simulink model "nn_plus"  (R2018b)
settings: Solver=VariableStepAuto  StartTime=0.0  StopTime=10.0  RelTol=1e-3
libraries: neural x265
(part 1 of 2)
settings Model: Creator=Mihail  LastModifiedBy=Mihail

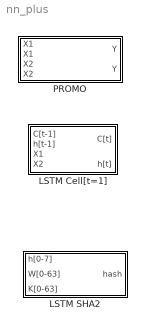
== system nn_plus ==
  LSTM Cell[t=1] : Subsystem
  LSTM SHA2 : Subsystem
  PROMO : Subsystem

== system nn_plus/LSTM Cell[t=1] ==
  note: LSTM Cell L1 (Block-Scheme)
  C[t-1] : Inport
  h[t-1] : Inport  Port=2
  X1 : Inport  Port=3
  X2 : Inport  Port=4
  Product : Product
  Product1 : Product
  Sum : Sum  Inputs=|++
  Sum1 : Sum  Inputs=|++
  Vector Concatenate : Concatenate  NumInputs=3
  logsig : neural/Transfer Functions/logsig
  logsig1 : neural/Transfer Functions/logsig
  logsig2 : neural/Transfer Functions/logsig
  tansig3 : neural/Transfer Functions/tansig
  tansig4 : neural/Transfer Functions/tansig
  C[t] : Outport
  h[t] : Outport  Port=2
  wires:
  h[t-1]/1 -> Vector Concatenate/1
  X1/1 -> Vector Concatenate/2
  X2/1 -> Vector Concatenate/3
  Vector Concatenate/1 -> logsig/1, logsig2/1, tansig3/1, logsig1/1
  C[t-1]/1 -> Sum/1
  logsig/1 -> Sum/2
  Sum/1 -> Sum1/1
  tansig3/1 -> Product/2
  logsig1/1 -> Product/1
  Product/1 -> Sum1/2
  logsig2/1 -> Product1/2
  Sum1/1 -> C[t]/1, tansig4/1
  tansig4/1 -> Product1/1
  Product1/1 -> h[t]/1

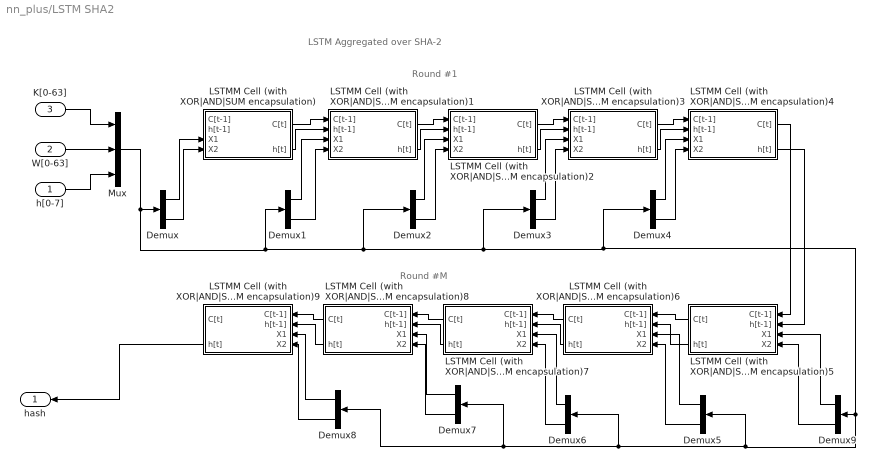
== system nn_plus/LSTM SHA2 ==
  note: Round #M
  note: Round #1
  note: LSTM Aggregated over SHA-2
  h[0-7] : Inport
  W[0-63] : Inport  Port=2
  K[0-63] : Inport  Port=3
  Demux{,1..9} (10 alike) : Demux  Outputs=2
  LSTMM Cell (with XOR|AND|SUM encapsulation) : Subsystem
  LSTMM Cell (with XOR|AND|SUM encapsulation)1 : Subsystem
  LSTMM Cell (with XOR|AND|SUM encapsulation)2 : Subsystem
  LSTMM Cell (with XOR|AND|SUM encapsulation)3 : Subsystem
  LSTMM Cell (with XOR|AND|SUM encapsulation)4 : Subsystem
  LSTMM Cell (with XOR|AND|SUM encapsulation)5 : Subsystem
  LSTMM Cell (with XOR|AND|SUM encapsulation)6 : Subsystem
  LSTMM Cell (with XOR|AND|SUM encapsulation)7 : Subsystem
  LSTMM Cell (with XOR|AND|SUM encapsulation)8 : Subsystem
  LSTMM Cell (with XOR|AND|SUM encapsulation)9 : Subsystem
  Mux : Mux  Inputs=3
  hash : Outport
  wires:
  Mux/1 -> Demux8/1, Demux7/1, Demux6/1, Demux5/1, Demux9/1, Demux4/1, Demux3/1, Demux2/1, Demux1/1, Demux/1
  Demux9/2 -> LSTMM Cell (with XOR|AND|SUM encapsulation)5/4(X2)
  LSTMM Cell (with XOR|AND|SUM encapsulation)7/2(h[t]) -> LSTMM Cell (with XOR|AND|SUM encapsulation)8/2(h[t-1])
  LSTMM Cell (with XOR|AND|SUM encapsulation)8/1(C[t]) -> LSTMM Cell (with XOR|AND|SUM encapsulation)9/1(C[t-1])
  LSTMM Cell (with XOR|AND|SUM encapsulation)5/2(h[t]) -> LSTMM Cell (with XOR|AND|SUM encapsulation)6/2(h[t-1])
  Demux5/1 -> LSTMM Cell (with XOR|AND|SUM encapsulation)6/3(X1)
  LSTMM Cell (with XOR|AND|SUM encapsulation)7/1(C[t]) -> LSTMM Cell (with XOR|AND|SUM encapsulation)8/1(C[t-1])
  Demux2/2 -> LSTMM Cell (with XOR|AND|SUM encapsulation)2/4(X2)
  Demux1/2 -> LSTMM Cell (with XOR|AND|SUM encapsulation)1/4(X2)
  Demux2/1 -> LSTMM Cell (with XOR|AND|SUM encapsulation)2/3(X1)
  Demux4/2 -> LSTMM Cell (with XOR|AND|SUM encapsulation)4/4(X2)
  Demux4/1 -> LSTMM Cell (with XOR|AND|SUM encapsulation)4/3(X1)
  Demux3/2 -> LSTMM Cell (with XOR|AND|SUM encapsulation)3/4(X2)
  Demux3/1 -> LSTMM Cell (with XOR|AND|SUM encapsulation)3/3(X1)
  Demux1/1 -> LSTMM Cell (with XOR|AND|SUM encapsulation)1/3(X1)
  LSTMM Cell (with XOR|AND|SUM encapsulation)2/2(h[t]) -> LSTMM Cell (with XOR|AND|SUM encapsulation)3/2(h[t-1])
  Demux7/1 -> LSTMM Cell (with XOR|AND|SUM encapsulation)8/3(X1)
  Demux/1 -> LSTMM Cell (with XOR|AND|SUM encapsulation)/3(X1)
  LSTMM Cell (with XOR|AND|SUM encapsulation)2/1(C[t]) -> LSTMM Cell (with XOR|AND|SUM encapsulation)3/1(C[t-1])
  Demux9/1 -> LSTMM Cell (with XOR|AND|SUM encapsulation)5/3(X1)
  Demux6/1 -> LSTMM Cell (with XOR|AND|SUM encapsulation)7/3(X1)
  Demux8/1 -> LSTMM Cell (with XOR|AND|SUM encapsulation)9/3(X1)
  Demux5/2 -> LSTMM Cell (with XOR|AND|SUM encapsulation)6/4(X2)
  Demux8/2 -> LSTMM Cell (with XOR|AND|SUM encapsulation)9/4(X2)
  LSTMM Cell (with XOR|AND|SUM encapsulation)8/2(h[t]) -> LSTMM Cell (with XOR|AND|SUM encapsulation)9/2(h[t-1])
  Demux7/2 -> LSTMM Cell (with XOR|AND|SUM encapsulation)8/4(X2)
  LSTMM Cell (with XOR|AND|SUM encapsulation)6/2(h[t]) -> LSTMM Cell (with XOR|AND|SUM encapsulation)7/2(h[t-1])
  Demux/2 -> LSTMM Cell (with XOR|AND|SUM encapsulation)/4(X2)
  K[0-63]/1 -> Mux/1
  LSTMM Cell (with XOR|AND|SUM encapsulation)/2(h[t]) -> LSTMM Cell (with XOR|AND|SUM encapsulation)1/2(h[t-1])
  LSTMM Cell (with XOR|AND|SUM encapsulation)1/2(h[t]) -> LSTMM Cell (with XOR|AND|SUM encapsulation)2/2(h[t-1])
  LSTMM Cell (with XOR|AND|SUM encapsulation)1/1(C[t]) -> LSTMM Cell (with XOR|AND|SUM encapsulation)2/1(C[t-1])
  LSTMM Cell (with XOR|AND|SUM encapsulation)9/2(h[t]) -> hash/1
  LSTMM Cell (with XOR|AND|SUM encapsulation)/1(C[t]) -> LSTMM Cell (with XOR|AND|SUM encapsulation)1/1(C[t-1])
  LSTMM Cell (with XOR|AND|SUM encapsulation)6/1(C[t]) -> LSTMM Cell (with XOR|AND|SUM encapsulation)7/1(C[t-1])
  LSTMM Cell (with XOR|AND|SUM encapsulation)3/1(C[t]) -> LSTMM Cell (with XOR|AND|SUM encapsulation)4/1(C[t-1])
  LSTMM Cell (with XOR|AND|SUM encapsulation)4/1(C[t]) -> LSTMM Cell (with XOR|AND|SUM encapsulation)5/1(C[t-1])
  W[0-63]/1 -> Mux/2
  Demux6/2 -> LSTMM Cell (with XOR|AND|SUM encapsulation)7/4(X2)
  LSTMM Cell (with XOR|AND|SUM encapsulation)4/2(h[t]) -> LSTMM Cell (with XOR|AND|SUM encapsulation)5/2(h[t-1])
  LSTMM Cell (with XOR|AND|SUM encapsulation)3/2(h[t]) -> LSTMM Cell (with XOR|AND|SUM encapsulation)4/2(h[t-1])
  h[0-7]/1 -> Mux/3
  LSTMM Cell (with XOR|AND|SUM encapsulation)5/1(C[t]) -> LSTMM Cell (with XOR|AND|SUM encapsulation)6/1(C[t-1])

== system nn_plus/PROMO ==
  note: SUM Overloaded
      | (Block-Scheme)
  note: SUM (As displayed)
  "X1 " : Inport
  X1 : Inport  Port=2
  X2 : Inport  Port=3
  "X2 " : Inport  Port=4
  Demux : Demux  Outputs=32
  Demux1 : Demux  Outputs=32
  Mux : Mux  Inputs=32
  SUM NN : Subsystem
  Sum : Sum  Inputs=|++
  Y : Outport
  "Y " : Outport  Port=2
  wires:
  Demux1/3 -> SUM NN/4(X2[t=1])
  Demux/32 -> SUM NN/7(X1[t=31])
  SUM NN/2(Y[t=1]) -> Mux/2
  SUM NN/1(Y[t=0]) -> Mux/1
  Demux/3 -> SUM NN/3(X1[t=1])
  Demux1/2 -> SUM NN/2(X2[t=0])
  SUM NN/4(Y[t=31]) -> Mux/32
  Demux1/32 -> SUM NN/8(X2[t=31])
  X1/1 -> Demux/1
  X2/1 -> Demux1/1
  "X2 "/1 -> Sum/2
  Sum/1 -> "Y "/1
  Mux/1 -> Y/1
  Demux/2 -> SUM NN/1(X1[t=0])
  "X1 "/1 -> Sum/1
  SUM NN/3(Y[t]) -> Mux/19

== system nn_plus/LSTM SHA2/LSTMM Cell (with XOR|AND|SUM encapsulation) ==
  note: LSTM Cell with LSTMM | XOR | AND NN (Used As Activation)
  C[t-1] : Inport
  h[t-1] : Inport  Port=2
  X1 : Inport  Port=3
  X2 : Inport  Port=4
  Demux : Demux  Outputs=2
  LSTM | XOR |AND (NN) : Subsystem
  Product : Product
  Product1 : Product
  Sum : Sum  Inputs=|++
  Sum1 : Sum  Inputs=|++
  Vector Concatenate : Concatenate  NumInputs=3
  logsig : neural/Transfer Functions/logsig
  logsig1 : neural/Transfer Functions/logsig
  tansig3 : neural/Transfer Functions/tansig
  tansig4 : neural/Transfer Functions/tansig
  C[t] : Outport
  h[t] : Outport  Port=2
  wires:
  h[t-1]/1 -> Vector Concatenate/1
  X1/1 -> Vector Concatenate/2
  X2/1 -> Vector Concatenate/3
  Vector Concatenate/1 -> logsig/1, Demux/1, tansig3/1, logsig1/1
  C[t-1]/1 -> Sum/1
  logsig/1 -> Sum/2
  Sum/1 -> Sum1/1
  tansig3/1 -> Product/2
  logsig1/1 -> Product/1
  Product/1 -> Sum1/2
  Sum1/1 -> C[t]/1, tansig4/1
  tansig4/1 -> Product1/1
  Product1/1 -> h[t]/1
  Demux/1 -> LSTM | XOR |AND (NN)/1(X1)
  Demux/2 -> LSTM | XOR |AND (NN)/2(X2)
  LSTM | XOR |AND (NN)/1(Y) -> Product1/2

== system nn_plus/LSTM SHA2/LSTMM Cell (with XOR|AND|SUM encapsulation)1 ==
  note: LSTM Cell with LSTMM | XOR | AND NN (Used As Activation)
  C[t-1] : Inport
  h[t-1] : Inport  Port=2
  X1 : Inport  Port=3
  X2 : Inport  Port=4
  Demux : Demux  Outputs=2
  LSTM | XOR |AND (NN) : Subsystem
  Product : Product
  Product1 : Product
  Sum : Sum  Inputs=|++
  Sum1 : Sum  Inputs=|++
  Vector Concatenate : Concatenate  NumInputs=3
  logsig : neural/Transfer Functions/logsig
  logsig1 : neural/Transfer Functions/logsig
  tansig3 : neural/Transfer Functions/tansig
  tansig4 : neural/Transfer Functions/tansig
  C[t] : Outport
  h[t] : Outport  Port=2
  wires:
  h[t-1]/1 -> Vector Concatenate/1
  X1/1 -> Vector Concatenate/2
  X2/1 -> Vector Concatenate/3
  Vector Concatenate/1 -> logsig/1, Demux/1, tansig3/1, logsig1/1
  C[t-1]/1 -> Sum/1
  logsig/1 -> Sum/2
  Sum/1 -> Sum1/1
  tansig3/1 -> Product/2
  logsig1/1 -> Product/1
  Product/1 -> Sum1/2
  Sum1/1 -> C[t]/1, tansig4/1
  tansig4/1 -> Product1/1
  Product1/1 -> h[t]/1
  Demux/1 -> LSTM | XOR |AND (NN)/1(X1)
  Demux/2 -> LSTM | XOR |AND (NN)/2(X2)
  LSTM | XOR |AND (NN)/1(Y) -> Product1/2

== system nn_plus/LSTM SHA2/LSTMM Cell (with XOR|AND|SUM encapsulation)2 ==
  note: LSTM Cell with LSTMM | XOR | AND NN (Used As Activation)
  C[t-1] : Inport
  h[t-1] : Inport  Port=2
  X1 : Inport  Port=3
  X2 : Inport  Port=4
  Demux : Demux  Outputs=2
  LSTM | XOR |AND (NN) : Subsystem
  Product : Product
  Product1 : Product
  Sum : Sum  Inputs=|++
  Sum1 : Sum  Inputs=|++
  Vector Concatenate : Concatenate  NumInputs=3
  logsig : neural/Transfer Functions/logsig
  logsig1 : neural/Transfer Functions/logsig
  tansig3 : neural/Transfer Functions/tansig
  tansig4 : neural/Transfer Functions/tansig
  C[t] : Outport
  h[t] : Outport  Port=2
  wires:
  h[t-1]/1 -> Vector Concatenate/1
  X1/1 -> Vector Concatenate/2
  X2/1 -> Vector Concatenate/3
  Vector Concatenate/1 -> logsig/1, Demux/1, tansig3/1, logsig1/1
  C[t-1]/1 -> Sum/1
  logsig/1 -> Sum/2
  Sum/1 -> Sum1/1
  tansig3/1 -> Product/2
  logsig1/1 -> Product/1
  Product/1 -> Sum1/2
  Sum1/1 -> C[t]/1, tansig4/1
  tansig4/1 -> Product1/1
  Product1/1 -> h[t]/1
  Demux/1 -> LSTM | XOR |AND (NN)/1(X1)
  Demux/2 -> LSTM | XOR |AND (NN)/2(X2)
  LSTM | XOR |AND (NN)/1(Y) -> Product1/2

== system nn_plus/LSTM SHA2/LSTMM Cell (with XOR|AND|SUM encapsulation)3 ==
  note: LSTM Cell with LSTMM | XOR | AND NN (Used As Activation)
  C[t-1] : Inport
  h[t-1] : Inport  Port=2
  X1 : Inport  Port=3
  X2 : Inport  Port=4
  Demux : Demux  Outputs=2
  LSTM | XOR |AND (NN) : Subsystem
  Product : Product
  Product1 : Product
  Sum : Sum  Inputs=|++
  Sum1 : Sum  Inputs=|++
  Vector Concatenate : Concatenate  NumInputs=3
  logsig : neural/Transfer Functions/logsig
  logsig1 : neural/Transfer Functions/logsig
  tansig3 : neural/Transfer Functions/tansig
  tansig4 : neural/Transfer Functions/tansig
  C[t] : Outport
  h[t] : Outport  Port=2
  wires:
  h[t-1]/1 -> Vector Concatenate/1
  X1/1 -> Vector Concatenate/2
  X2/1 -> Vector Concatenate/3
  Vector Concatenate/1 -> logsig/1, Demux/1, tansig3/1, logsig1/1
  C[t-1]/1 -> Sum/1
  logsig/1 -> Sum/2
  Sum/1 -> Sum1/1
  tansig3/1 -> Product/2
  logsig1/1 -> Product/1
  Product/1 -> Sum1/2
  Sum1/1 -> C[t]/1, tansig4/1
  tansig4/1 -> Product1/1
  Product1/1 -> h[t]/1
  Demux/1 -> LSTM | XOR |AND (NN)/1(X1)
  Demux/2 -> LSTM | XOR |AND (NN)/2(X2)
  LSTM | XOR |AND (NN)/1(Y) -> Product1/2

== system nn_plus/LSTM SHA2/LSTMM Cell (with XOR|AND|SUM encapsulation)4 ==
  note: LSTM Cell with LSTMM | XOR | AND NN (Used As Activation)
  C[t-1] : Inport
  h[t-1] : Inport  Port=2
  X1 : Inport  Port=3
  X2 : Inport  Port=4
  Demux : Demux  Outputs=2
  LSTM | XOR |AND (NN) : Subsystem
  Product : Product
  Product1 : Product
  Sum : Sum  Inputs=|++
  Sum1 : Sum  Inputs=|++
  Vector Concatenate : Concatenate  NumInputs=3
  logsig : neural/Transfer Functions/logsig
  logsig1 : neural/Transfer Functions/logsig
  tansig3 : neural/Transfer Functions/tansig
  tansig4 : neural/Transfer Functions/tansig
  C[t] : Outport
  h[t] : Outport  Port=2
  wires:
  h[t-1]/1 -> Vector Concatenate/1
  X1/1 -> Vector Concatenate/2
  X2/1 -> Vector Concatenate/3
  Vector Concatenate/1 -> logsig/1, Demux/1, tansig3/1, logsig1/1
  C[t-1]/1 -> Sum/1
  logsig/1 -> Sum/2
  Sum/1 -> Sum1/1
  tansig3/1 -> Product/2
  logsig1/1 -> Product/1
  Product/1 -> Sum1/2
  Sum1/1 -> C[t]/1, tansig4/1
  tansig4/1 -> Product1/1
  Product1/1 -> h[t]/1
  Demux/1 -> LSTM | XOR |AND (NN)/1(X1)
  Demux/2 -> LSTM | XOR |AND (NN)/2(X2)
  LSTM | XOR |AND (NN)/1(Y) -> Product1/2

== system nn_plus/LSTM SHA2/LSTMM Cell (with XOR|AND|SUM encapsulation)5 ==
  note: LSTM Cell with LSTMM | XOR | AND NN (Used As Activation)
  C[t-1] : Inport
  h[t-1] : Inport  Port=2
  X1 : Inport  Port=3
  X2 : Inport  Port=4
  Demux : Demux  Outputs=2
  LSTM | XOR |AND (NN) : Subsystem
  Product : Product
  Product1 : Product
  Sum : Sum  Inputs=|++
  Sum1 : Sum  Inputs=|++
  Vector Concatenate : Concatenate  NumInputs=3
  logsig : neural/Transfer Functions/logsig
  logsig1 : neural/Transfer Functions/logsig
  tansig3 : neural/Transfer Functions/tansig
  tansig4 : neural/Transfer Functions/tansig
  C[t] : Outport
  h[t] : Outport  Port=2
  wires:
  h[t-1]/1 -> Vector Concatenate/1
  X1/1 -> Vector Concatenate/2
  X2/1 -> Vector Concatenate/3
  Vector Concatenate/1 -> logsig/1, Demux/1, tansig3/1, logsig1/1
  C[t-1]/1 -> Sum/1
  logsig/1 -> Sum/2
  Sum/1 -> Sum1/1
  tansig3/1 -> Product/2
  logsig1/1 -> Product/1
  Product/1 -> Sum1/2
  Sum1/1 -> C[t]/1, tansig4/1
  tansig4/1 -> Product1/1
  Product1/1 -> h[t]/1
  Demux/1 -> LSTM | XOR |AND (NN)/1(X1)
  Demux/2 -> LSTM | XOR |AND (NN)/2(X2)
  LSTM | XOR |AND (NN)/1(Y) -> Product1/2

== system nn_plus/LSTM SHA2/LSTMM Cell (with XOR|AND|SUM encapsulation)6 ==
  note: LSTM Cell with LSTMM | XOR | AND NN (Used As Activation)
  C[t-1] : Inport
  h[t-1] : Inport  Port=2
  X1 : Inport  Port=3
  X2 : Inport  Port=4
  Demux : Demux  Outputs=2
  LSTM | XOR |AND (NN) : Subsystem
  Product : Product
  Product1 : Product
  Sum : Sum  Inputs=|++
  Sum1 : Sum  Inputs=|++
  Vector Concatenate : Concatenate  NumInputs=3
  logsig : neural/Transfer Functions/logsig
  logsig1 : neural/Transfer Functions/logsig
  tansig3 : neural/Transfer Functions/tansig
  tansig4 : neural/Transfer Functions/tansig
  C[t] : Outport
  h[t] : Outport  Port=2
  wires:
  h[t-1]/1 -> Vector Concatenate/1
  X1/1 -> Vector Concatenate/2
  X2/1 -> Vector Concatenate/3
  Vector Concatenate/1 -> logsig/1, Demux/1, tansig3/1, logsig1/1
  C[t-1]/1 -> Sum/1
  logsig/1 -> Sum/2
  Sum/1 -> Sum1/1
  tansig3/1 -> Product/2
  logsig1/1 -> Product/1
  Product/1 -> Sum1/2
  Sum1/1 -> C[t]/1, tansig4/1
  tansig4/1 -> Product1/1
  Product1/1 -> h[t]/1
  Demux/1 -> LSTM | XOR |AND (NN)/1(X1)
  Demux/2 -> LSTM | XOR |AND (NN)/2(X2)
  LSTM | XOR |AND (NN)/1(Y) -> Product1/2

== system nn_plus/LSTM SHA2/LSTMM Cell (with XOR|AND|SUM encapsulation)7 ==
  note: LSTM Cell with LSTMM | XOR | AND NN (Used As Activation)
  C[t-1] : Inport
  h[t-1] : Inport  Port=2
  X1 : Inport  Port=3
  X2 : Inport  Port=4
  Demux : Demux  Outputs=2
  LSTM | XOR |AND (NN) : Subsystem
  Product : Product
  Product1 : Product
  Sum : Sum  Inputs=|++
  Sum1 : Sum  Inputs=|++
  Vector Concatenate : Concatenate  NumInputs=3
  logsig : neural/Transfer Functions/logsig
  logsig1 : neural/Transfer Functions/logsig
  tansig3 : neural/Transfer Functions/tansig
  tansig4 : neural/Transfer Functions/tansig
  C[t] : Outport
  h[t] : Outport  Port=2
  wires:
  h[t-1]/1 -> Vector Concatenate/1
  X1/1 -> Vector Concatenate/2
  X2/1 -> Vector Concatenate/3
  Vector Concatenate/1 -> logsig/1, Demux/1, tansig3/1, logsig1/1
  C[t-1]/1 -> Sum/1
  logsig/1 -> Sum/2
  Sum/1 -> Sum1/1
  tansig3/1 -> Product/2
  logsig1/1 -> Product/1
  Product/1 -> Sum1/2
  Sum1/1 -> C[t]/1, tansig4/1
  tansig4/1 -> Product1/1
  Product1/1 -> h[t]/1
  Demux/1 -> LSTM | XOR |AND (NN)/1(X1)
  Demux/2 -> LSTM | XOR |AND (NN)/2(X2)
  LSTM | XOR |AND (NN)/1(Y) -> Product1/2

== system nn_plus/LSTM SHA2/LSTMM Cell (with XOR|AND|SUM encapsulation)8 ==
  note: LSTM Cell with LSTMM | XOR | AND NN (Used As Activation)
  C[t-1] : Inport
  h[t-1] : Inport  Port=2
  X1 : Inport  Port=3
  X2 : Inport  Port=4
  Demux : Demux  Outputs=2
  LSTM | XOR |AND (NN) : Subsystem
  Product : Product
  Product1 : Product
  Sum : Sum  Inputs=|++
  Sum1 : Sum  Inputs=|++
  Vector Concatenate : Concatenate  NumInputs=3
  logsig : neural/Transfer Functions/logsig
  logsig1 : neural/Transfer Functions/logsig
  tansig3 : neural/Transfer Functions/tansig
  tansig4 : neural/Transfer Functions/tansig
  C[t] : Outport
  h[t] : Outport  Port=2
  wires:
  h[t-1]/1 -> Vector Concatenate/1
  X1/1 -> Vector Concatenate/2
  X2/1 -> Vector Concatenate/3
  Vector Concatenate/1 -> logsig/1, Demux/1, tansig3/1, logsig1/1
  C[t-1]/1 -> Sum/1
  logsig/1 -> Sum/2
  Sum/1 -> Sum1/1
  tansig3/1 -> Product/2
  logsig1/1 -> Product/1
  Product/1 -> Sum1/2
  Sum1/1 -> C[t]/1, tansig4/1
  tansig4/1 -> Product1/1
  Product1/1 -> h[t]/1
  Demux/1 -> LSTM | XOR |AND (NN)/1(X1)
  Demux/2 -> LSTM | XOR |AND (NN)/2(X2)
  LSTM | XOR |AND (NN)/1(Y) -> Product1/2

== system nn_plus/LSTM SHA2/LSTMM Cell (with XOR|AND|SUM encapsulation)9 ==
  note: LSTM Cell with LSTMM | XOR | AND NN (Used As Activation)
  C[t-1] : Inport
  h[t-1] : Inport  Port=2
  X1 : Inport  Port=3
  X2 : Inport  Port=4
  Demux : Demux  Outputs=2
  LSTM | XOR |AND (NN) : Subsystem
  Product : Product
  Product1 : Product
  Sum : Sum  Inputs=|++
  Sum1 : Sum  Inputs=|++
  Vector Concatenate : Concatenate  NumInputs=3
  logsig : neural/Transfer Functions/logsig
  logsig1 : neural/Transfer Functions/logsig
  tansig3 : neural/Transfer Functions/tansig
  tansig4 : neural/Transfer Functions/tansig
  C[t] : Outport
  h[t] : Outport  Port=2
  wires:
  h[t-1]/1 -> Vector Concatenate/1
  X1/1 -> Vector Concatenate/2
  X2/1 -> Vector Concatenate/3
  Vector Concatenate/1 -> logsig/1, Demux/1, tansig3/1, logsig1/1
  C[t-1]/1 -> Sum/1
  logsig/1 -> Sum/2
  Sum/1 -> Sum1/1
  tansig3/1 -> Product/2
  logsig1/1 -> Product/1
  Product/1 -> Sum1/2
  Sum1/1 -> C[t]/1, tansig4/1
  tansig4/1 -> Product1/1
  Product1/1 -> h[t]/1
  Demux/1 -> LSTM | XOR |AND (NN)/1(X1)
  Demux/2 -> LSTM | XOR |AND (NN)/2(X2)
  LSTM | XOR |AND (NN)/1(Y) -> Product1/2

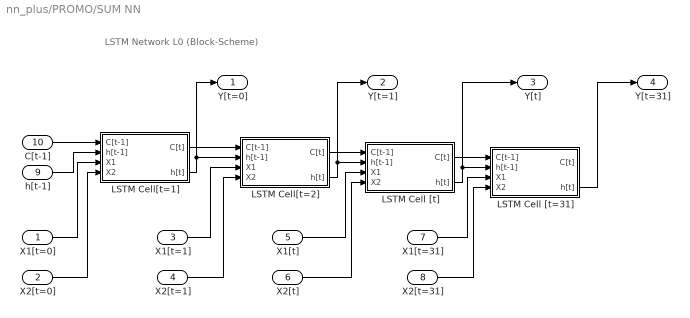
== system nn_plus/PROMO/SUM NN ==
  note: LSTM Network L0 (Block-Scheme)
  X1[t=0] : Inport
  X2[t=0] : Inport  Port=2
  X1[t=1] : Inport  Port=3
  X2[t=1] : Inport  Port=4
  X1[t] : Inport  Port=5
  X2[t] : Inport  Port=6
  X1[t=31] : Inport  Port=7
  X2[t=31] : Inport  Port=8
  h[t-1] : Inport  Port=9
  C[t-1] : Inport  Port=10
  LSTM Cell [t=31] : Subsystem
  LSTM Cell [t] : Subsystem
  LSTM Cell[t=1] : Subsystem
  LSTM Cell[t=2] : Subsystem
  Y[t=0] : Outport
  Y[t=1] : Outport  Port=2
  Y[t] : Outport  Port=3
  Y[t=31] : Outport  Port=4
  wires:
  C[t-1]/1 -> LSTM Cell[t=1]/1(C[t-1])
  h[t-1]/1 -> LSTM Cell[t=1]/2(h[t-1])
  LSTM Cell[t=1]/1(C[t]) -> LSTM Cell[t=2]/1(C[t-1])
  LSTM Cell[t=1]/2(h[t]) -> Y[t=0]/1, LSTM Cell[t=2]/2(h[t-1])
  X1[t=0]/1 -> LSTM Cell[t=1]/3(X1)
  X2[t=0]/1 -> LSTM Cell[t=1]/4(X2)
  X1[t=1]/1 -> LSTM Cell[t=2]/3(X1)
  X2[t=1]/1 -> LSTM Cell[t=2]/4(X2)
  LSTM Cell[t=2]/1(C[t]) -> LSTM Cell [t]/1(C[t-1])
  LSTM Cell[t=2]/2(h[t]) -> Y[t=1]/1, LSTM Cell [t]/2(h[t-1])
  LSTM Cell [t]/1(C[t]) -> LSTM Cell [t=31]/1(C[t-1])
  X2[t]/1 -> LSTM Cell [t]/4(X2)
  X1[t]/1 -> LSTM Cell [t]/3(X1)
  X1[t=31]/1 -> LSTM Cell [t=31]/3(X1)
  X2[t=31]/1 -> LSTM Cell [t=31]/4(X2)
  LSTM Cell [t=31]/2(h[t]) -> Y[t=31]/1
  LSTM Cell [t]/2(h[t]) -> Y[t]/1, LSTM Cell [t=31]/2(h[t-1])

== system nn_plus/LSTM SHA2/LSTMM Cell (with XOR|AND|SUM encapsulation)/LSTM | XOR |AND (NN) ==
  note: SUM Overloaded
      | (Block-Scheme)
  X1 : Inport
  X2 : Inport  Port=2
  Demux : Demux  Outputs=32
  Demux1 : Demux  Outputs=32
  Mux : Mux  Inputs=32
  SUM NN : Subsystem
  Y : Outport
  wires:
  Demux1/3 -> SUM NN/4(X2[t=1])
  Demux/32 -> SUM NN/7(X1[t=31])
  SUM NN/2(Y[t=1]) -> Mux/2
  SUM NN/1(Y[t=0]) -> Mux/1
  Demux/3 -> SUM NN/3(X1[t=1])
  Demux1/2 -> SUM NN/2(X2[t=0])
  SUM NN/4(Y[t=31]) -> Mux/32
  Demux1/32 -> SUM NN/8(X2[t=31])
  X1/1 -> Demux/1
  X2/1 -> Demux1/1
  Mux/1 -> Y/1
  Demux/2 -> SUM NN/1(X1[t=0])
  SUM NN/3(Y[t]) -> Mux/19

== system nn_plus/LSTM SHA2/LSTMM Cell (with XOR|AND|SUM encapsulation)1/LSTM | XOR |AND (NN) ==
  note: SUM Overloaded
      | (Block-Scheme)
  X1 : Inport
  X2 : Inport  Port=2
  Demux : Demux  Outputs=32
  Demux1 : Demux  Outputs=32
  Mux : Mux  Inputs=32
  SUM NN : Subsystem
  Y : Outport
  wires:
  Demux1/3 -> SUM NN/4(X2[t=1])
  Demux/32 -> SUM NN/7(X1[t=31])
  SUM NN/2(Y[t=1]) -> Mux/2
  SUM NN/1(Y[t=0]) -> Mux/1
  Demux/3 -> SUM NN/3(X1[t=1])
  Demux1/2 -> SUM NN/2(X2[t=0])
  SUM NN/4(Y[t=31]) -> Mux/32
  Demux1/32 -> SUM NN/8(X2[t=31])
  X1/1 -> Demux/1
  X2/1 -> Demux1/1
  Mux/1 -> Y/1
  Demux/2 -> SUM NN/1(X1[t=0])
  SUM NN/3(Y[t]) -> Mux/19

== system nn_plus/LSTM SHA2/LSTMM Cell (with XOR|AND|SUM encapsulation)2/LSTM | XOR |AND (NN) ==
  note: SUM Overloaded
      | (Block-Scheme)
  X1 : Inport
  X2 : Inport  Port=2
  Demux : Demux  Outputs=32
  Demux1 : Demux  Outputs=32
  Mux : Mux  Inputs=32
  SUM NN : Subsystem
  Y : Outport
  wires:
  Demux1/3 -> SUM NN/4(X2[t=1])
  Demux/32 -> SUM NN/7(X1[t=31])
  SUM NN/2(Y[t=1]) -> Mux/2
  SUM NN/1(Y[t=0]) -> Mux/1
  Demux/3 -> SUM NN/3(X1[t=1])
  Demux1/2 -> SUM NN/2(X2[t=0])
  SUM NN/4(Y[t=31]) -> Mux/32
  Demux1/32 -> SUM NN/8(X2[t=31])
  X1/1 -> Demux/1
  X2/1 -> Demux1/1
  Mux/1 -> Y/1
  Demux/2 -> SUM NN/1(X1[t=0])
  SUM NN/3(Y[t]) -> Mux/19

== system nn_plus/LSTM SHA2/LSTMM Cell (with XOR|AND|SUM encapsulation)3/LSTM | XOR |AND (NN) ==
  note: SUM Overloaded
      | (Block-Scheme)
  X1 : Inport
  X2 : Inport  Port=2
  Demux : Demux  Outputs=32
  Demux1 : Demux  Outputs=32
  Mux : Mux  Inputs=32
  SUM NN : Subsystem
  Y : Outport
  wires:
  Demux1/3 -> SUM NN/4(X2[t=1])
  Demux/32 -> SUM NN/7(X1[t=31])
  SUM NN/2(Y[t=1]) -> Mux/2
  SUM NN/1(Y[t=0]) -> Mux/1
  Demux/3 -> SUM NN/3(X1[t=1])
  Demux1/2 -> SUM NN/2(X2[t=0])
  SUM NN/4(Y[t=31]) -> Mux/32
  Demux1/32 -> SUM NN/8(X2[t=31])
  X1/1 -> Demux/1
  X2/1 -> Demux1/1
  Mux/1 -> Y/1
  Demux/2 -> SUM NN/1(X1[t=0])
  SUM NN/3(Y[t]) -> Mux/19

== system nn_plus/LSTM SHA2/LSTMM Cell (with XOR|AND|SUM encapsulation)4/LSTM | XOR |AND (NN) ==
  note: SUM Overloaded
      | (Block-Scheme)
  X1 : Inport
  X2 : Inport  Port=2
  Demux : Demux  Outputs=32
  Demux1 : Demux  Outputs=32
  Mux : Mux  Inputs=32
  SUM NN : Subsystem
  Y : Outport
  wires:
  Demux1/3 -> SUM NN/4(X2[t=1])
  Demux/32 -> SUM NN/7(X1[t=31])
  SUM NN/2(Y[t=1]) -> Mux/2
  SUM NN/1(Y[t=0]) -> Mux/1
  Demux/3 -> SUM NN/3(X1[t=1])
  Demux1/2 -> SUM NN/2(X2[t=0])
  SUM NN/4(Y[t=31]) -> Mux/32
  Demux1/32 -> SUM NN/8(X2[t=31])
  X1/1 -> Demux/1
  X2/1 -> Demux1/1
  Mux/1 -> Y/1
  Demux/2 -> SUM NN/1(X1[t=0])
  SUM NN/3(Y[t]) -> Mux/19

== system nn_plus/LSTM SHA2/LSTMM Cell (with XOR|AND|SUM encapsulation)5/LSTM | XOR |AND (NN) ==
  note: SUM Overloaded
      | (Block-Scheme)
  X1 : Inport
  X2 : Inport  Port=2
  Demux : Demux  Outputs=32
  Demux1 : Demux  Outputs=32
  Mux : Mux  Inputs=32
  SUM NN : Subsystem
  Y : Outport
  wires:
  Demux1/3 -> SUM NN/4(X2[t=1])
  Demux/32 -> SUM NN/7(X1[t=31])
  SUM NN/2(Y[t=1]) -> Mux/2
  SUM NN/1(Y[t=0]) -> Mux/1
  Demux/3 -> SUM NN/3(X1[t=1])
  Demux1/2 -> SUM NN/2(X2[t=0])
  SUM NN/4(Y[t=31]) -> Mux/32
  Demux1/32 -> SUM NN/8(X2[t=31])
  X1/1 -> Demux/1
  X2/1 -> Demux1/1
  Mux/1 -> Y/1
  Demux/2 -> SUM NN/1(X1[t=0])
  SUM NN/3(Y[t]) -> Mux/19

== system nn_plus/LSTM SHA2/LSTMM Cell (with XOR|AND|SUM encapsulation)6/LSTM | XOR |AND (NN) ==
  note: SUM Overloaded
      | (Block-Scheme)
  X1 : Inport
  X2 : Inport  Port=2
  Demux : Demux  Outputs=32
  Demux1 : Demux  Outputs=32
  Mux : Mux  Inputs=32
  SUM NN : Subsystem
  Y : Outport
  wires:
  Demux1/3 -> SUM NN/4(X2[t=1])
  Demux/32 -> SUM NN/7(X1[t=31])
  SUM NN/2(Y[t=1]) -> Mux/2
  SUM NN/1(Y[t=0]) -> Mux/1
  Demux/3 -> SUM NN/3(X1[t=1])
  Demux1/2 -> SUM NN/2(X2[t=0])
  SUM NN/4(Y[t=31]) -> Mux/32
  Demux1/32 -> SUM NN/8(X2[t=31])
  X1/1 -> Demux/1
  X2/1 -> Demux1/1
  Mux/1 -> Y/1
  Demux/2 -> SUM NN/1(X1[t=0])
  SUM NN/3(Y[t]) -> Mux/19

== system nn_plus/LSTM SHA2/LSTMM Cell (with XOR|AND|SUM encapsulation)7/LSTM | XOR |AND (NN) ==
  note: SUM Overloaded
      | (Block-Scheme)
  X1 : Inport
  X2 : Inport  Port=2
  Demux : Demux  Outputs=32
  Demux1 : Demux  Outputs=32
  Mux : Mux  Inputs=32
  SUM NN : Subsystem
  Y : Outport
  wires:
  Demux1/3 -> SUM NN/4(X2[t=1])
  Demux/32 -> SUM NN/7(X1[t=31])
  SUM NN/2(Y[t=1]) -> Mux/2
  SUM NN/1(Y[t=0]) -> Mux/1
  Demux/3 -> SUM NN/3(X1[t=1])
  Demux1/2 -> SUM NN/2(X2[t=0])
  SUM NN/4(Y[t=31]) -> Mux/32
  Demux1/32 -> SUM NN/8(X2[t=31])
  X1/1 -> Demux/1
  X2/1 -> Demux1/1
  Mux/1 -> Y/1
  Demux/2 -> SUM NN/1(X1[t=0])
  SUM NN/3(Y[t]) -> Mux/19

== system nn_plus/LSTM SHA2/LSTMM Cell (with XOR|AND|SUM encapsulation)8/LSTM | XOR |AND (NN) ==
  note: SUM Overloaded
      | (Block-Scheme)
  X1 : Inport
  X2 : Inport  Port=2
  Demux : Demux  Outputs=32
  Demux1 : Demux  Outputs=32
  Mux : Mux  Inputs=32
  SUM NN : Subsystem
  Y : Outport
  wires:
  Demux1/3 -> SUM NN/4(X2[t=1])
  Demux/32 -> SUM NN/7(X1[t=31])
  SUM NN/2(Y[t=1]) -> Mux/2
  SUM NN/1(Y[t=0]) -> Mux/1
  Demux/3 -> SUM NN/3(X1[t=1])
  Demux1/2 -> SUM NN/2(X2[t=0])
  SUM NN/4(Y[t=31]) -> Mux/32
  Demux1/32 -> SUM NN/8(X2[t=31])
  X1/1 -> Demux/1
  X2/1 -> Demux1/1
  Mux/1 -> Y/1
  Demux/2 -> SUM NN/1(X1[t=0])
  SUM NN/3(Y[t]) -> Mux/19

== system nn_plus/LSTM SHA2/LSTMM Cell (with XOR|AND|SUM encapsulation)9/LSTM | XOR |AND (NN) ==
  note: SUM Overloaded
      | (Block-Scheme)
  X1 : Inport
  X2 : Inport  Port=2
  Demux : Demux  Outputs=32
  Demux1 : Demux  Outputs=32
  Mux : Mux  Inputs=32
  SUM NN : Subsystem
  Y : Outport
  wires:
  Demux1/3 -> SUM NN/4(X2[t=1])
  Demux/32 -> SUM NN/7(X1[t=31])
  SUM NN/2(Y[t=1]) -> Mux/2
  SUM NN/1(Y[t=0]) -> Mux/1
  Demux/3 -> SUM NN/3(X1[t=1])
  Demux1/2 -> SUM NN/2(X2[t=0])
  SUM NN/4(Y[t=31]) -> Mux/32
  Demux1/32 -> SUM NN/8(X2[t=31])
  X1/1 -> Demux/1
  X2/1 -> Demux1/1
  Mux/1 -> Y/1
  Demux/2 -> SUM NN/1(X1[t=0])
  SUM NN/3(Y[t]) -> Mux/19

== system nn_plus/PROMO/SUM NN/LSTM Cell [t=31] ==
  C[t-1] : Inport
  h[t-1] : Inport  Port=2
  X1 : Inport  Port=3
  X2 : Inport  Port=4
  Product : Product
  Product1 : Product
  Sum : Sum  Inputs=|++
  Sum1 : Sum  Inputs=|++
  Vector Concatenate : Concatenate  NumInputs=3
  logsig : neural/Transfer Functions/logsig
  logsig1 : neural/Transfer Functions/logsig
  logsig2 : neural/Transfer Functions/logsig
  tansig3 : neural/Transfer Functions/tansig
  tansig4 : neural/Transfer Functions/tansig
  C[t] : Outport
  h[t] : Outport  Port=2
  wires:
  h[t-1]/1 -> Vector Concatenate/1
  X1/1 -> Vector Concatenate/2
  X2/1 -> Vector Concatenate/3
  Vector Concatenate/1 -> tansig3/1, logsig2/1, logsig1/1, logsig/1
  C[t-1]/1 -> Sum/1
  logsig/1 -> Sum/2
  Sum/1 -> Sum1/1
  tansig3/1 -> Product/2
  logsig1/1 -> Product/1
  Product/1 -> Sum1/2
  logsig2/1 -> Product1/2
  Sum1/1 -> C[t]/1, tansig4/1
  tansig4/1 -> Product1/1
  Product1/1 -> h[t]/1

== system nn_plus/PROMO/SUM NN/LSTM Cell [t] ==
  C[t-1] : Inport
  h[t-1] : Inport  Port=2
  X1 : Inport  Port=3
  X2 : Inport  Port=4
  Product : Product
  Product1 : Product
  Sum : Sum  Inputs=|++
  Sum1 : Sum  Inputs=|++
  Vector Concatenate : Concatenate  NumInputs=3
  logsig : neural/Transfer Functions/logsig
  logsig1 : neural/Transfer Functions/logsig
  logsig2 : neural/Transfer Functions/logsig
  tansig3 : neural/Transfer Functions/tansig
  tansig4 : neural/Transfer Functions/tansig
  C[t] : Outport
  h[t] : Outport  Port=2
  wires:
  h[t-1]/1 -> Vector Concatenate/1
  X1/1 -> Vector Concatenate/2
  X2/1 -> Vector Concatenate/3
  Vector Concatenate/1 -> tansig3/1, logsig2/1, logsig1/1, logsig/1
  C[t-1]/1 -> Sum/1
  logsig/1 -> Sum/2
  Sum/1 -> Sum1/1
  tansig3/1 -> Product/2
  logsig1/1 -> Product/1
  Product/1 -> Sum1/2
  logsig2/1 -> Product1/2
  Sum1/1 -> C[t]/1, tansig4/1
  tansig4/1 -> Product1/1
  Product1/1 -> h[t]/1

== system nn_plus/PROMO/SUM NN/LSTM Cell[t=1] ==
  note: LSTM Cell L1 (Block-Scheme)
  C[t-1] : Inport
  h[t-1] : Inport  Port=2
  X1 : Inport  Port=3
  X2 : Inport  Port=4
  Product : Product
  Product1 : Product
  Sum : Sum  Inputs=|++
  Sum1 : Sum  Inputs=|++
  Vector Concatenate : Concatenate  NumInputs=3
  logsig : neural/Transfer Functions/logsig
  logsig1 : neural/Transfer Functions/logsig
  logsig2 : neural/Transfer Functions/logsig
  tansig3 : neural/Transfer Functions/tansig
  tansig4 : neural/Transfer Functions/tansig
  C[t] : Outport
  h[t] : Outport  Port=2
  wires:
  h[t-1]/1 -> Vector Concatenate/1
  X1/1 -> Vector Concatenate/2
  X2/1 -> Vector Concatenate/3
  Vector Concatenate/1 -> logsig/1, logsig2/1, tansig3/1, logsig1/1
  C[t-1]/1 -> Sum/1
  logsig/1 -> Sum/2
  Sum/1 -> Sum1/1
  tansig3/1 -> Product/2
  logsig1/1 -> Product/1
  Product/1 -> Sum1/2
  logsig2/1 -> Product1/2
  Sum1/1 -> C[t]/1, tansig4/1
  tansig4/1 -> Product1/1
  Product1/1 -> h[t]/1

== system nn_plus/PROMO/SUM NN/LSTM Cell[t=2] ==
  C[t-1] : Inport
  h[t-1] : Inport  Port=2
  X1 : Inport  Port=3
  X2 : Inport  Port=4
  Product : Product
  Product1 : Product
  Sum : Sum  Inputs=|++
  Sum1 : Sum  Inputs=|++
  Vector Concatenate : Concatenate  NumInputs=3
  logsig : neural/Transfer Functions/logsig
  logsig1 : neural/Transfer Functions/logsig
  logsig2 : neural/Transfer Functions/logsig
  tansig3 : neural/Transfer Functions/tansig
  tansig4 : neural/Transfer Functions/tansig
  C[t] : Outport
  h[t] : Outport  Port=2
  wires:
  h[t-1]/1 -> Vector Concatenate/1
  X1/1 -> Vector Concatenate/2
  X2/1 -> Vector Concatenate/3
  Vector Concatenate/1 -> tansig3/1, logsig2/1, logsig1/1, logsig/1
  C[t-1]/1 -> Sum/1
  logsig/1 -> Sum/2
  Sum/1 -> Sum1/1
  tansig3/1 -> Product/2
  logsig1/1 -> Product/1
  Product/1 -> Sum1/2
  logsig2/1 -> Product1/2
  Sum1/1 -> C[t]/1, tansig4/1
  tansig4/1 -> Product1/1
  Product1/1 -> h[t]/1

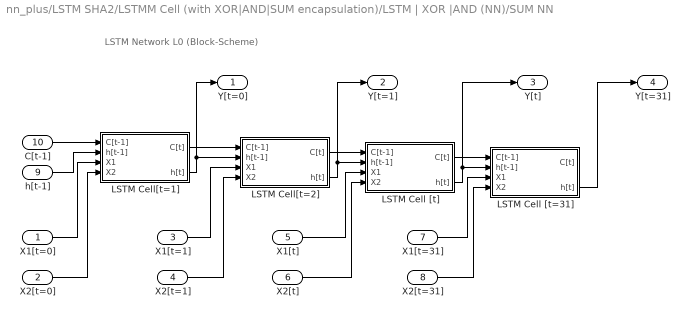
== system nn_plus/LSTM SHA2/LSTMM Cell (with XOR|AND|SUM encapsulation)/LSTM | XOR |AND (NN)/SUM NN ==
  note: LSTM Network L0 (Block-Scheme)
  X1[t=0] : Inport
  X2[t=0] : Inport  Port=2
  X1[t=1] : Inport  Port=3
  X2[t=1] : Inport  Port=4
  X1[t] : Inport  Port=5
  X2[t] : Inport  Port=6
  X1[t=31] : Inport  Port=7
  X2[t=31] : Inport  Port=8
  h[t-1] : Inport  Port=9
  C[t-1] : Inport  Port=10
  LSTM Cell [t=31] : Subsystem
  LSTM Cell [t] : Subsystem
  LSTM Cell[t=1] : Subsystem
  LSTM Cell[t=2] : Subsystem
  Y[t=0] : Outport
  Y[t=1] : Outport  Port=2
  Y[t] : Outport  Port=3
  Y[t=31] : Outport  Port=4
  wires:
  C[t-1]/1 -> LSTM Cell[t=1]/1(C[t-1])
  h[t-1]/1 -> LSTM Cell[t=1]/2(h[t-1])
  LSTM Cell[t=1]/1(C[t]) -> LSTM Cell[t=2]/1(C[t-1])
  LSTM Cell[t=1]/2(h[t]) -> Y[t=0]/1, LSTM Cell[t=2]/2(h[t-1])
  X1[t=0]/1 -> LSTM Cell[t=1]/3(X1)
  X2[t=0]/1 -> LSTM Cell[t=1]/4(X2)
  X1[t=1]/1 -> LSTM Cell[t=2]/3(X1)
  X2[t=1]/1 -> LSTM Cell[t=2]/4(X2)
  LSTM Cell[t=2]/1(C[t]) -> LSTM Cell [t]/1(C[t-1])
  LSTM Cell[t=2]/2(h[t]) -> Y[t=1]/1, LSTM Cell [t]/2(h[t-1])
  LSTM Cell [t]/1(C[t]) -> LSTM Cell [t=31]/1(C[t-1])
  X2[t]/1 -> LSTM Cell [t]/4(X2)
  X1[t]/1 -> LSTM Cell [t]/3(X1)
  X1[t=31]/1 -> LSTM Cell [t=31]/3(X1)
  X2[t=31]/1 -> LSTM Cell [t=31]/4(X2)
  LSTM Cell [t=31]/2(h[t]) -> Y[t=31]/1
  LSTM Cell [t]/2(h[t]) -> Y[t]/1, LSTM Cell [t=31]/2(h[t-1])

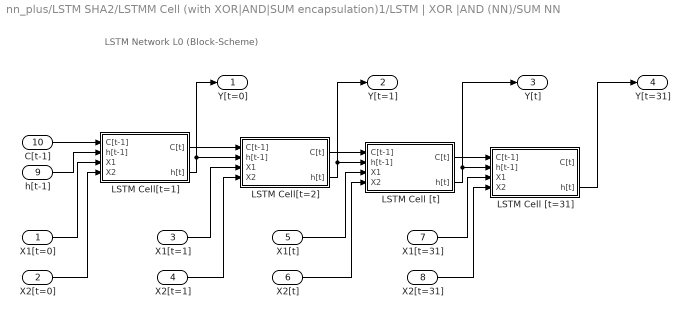
== system nn_plus/LSTM SHA2/LSTMM Cell (with XOR|AND|SUM encapsulation)1/LSTM | XOR |AND (NN)/SUM NN ==
  note: LSTM Network L0 (Block-Scheme)
  X1[t=0] : Inport
  X2[t=0] : Inport  Port=2
  X1[t=1] : Inport  Port=3
  X2[t=1] : Inport  Port=4
  X1[t] : Inport  Port=5
  X2[t] : Inport  Port=6
  X1[t=31] : Inport  Port=7
  X2[t=31] : Inport  Port=8
  h[t-1] : Inport  Port=9
  C[t-1] : Inport  Port=10
  LSTM Cell [t=31] : Subsystem
  LSTM Cell [t] : Subsystem
  LSTM Cell[t=1] : Subsystem
  LSTM Cell[t=2] : Subsystem
  Y[t=0] : Outport
  Y[t=1] : Outport  Port=2
  Y[t] : Outport  Port=3
  Y[t=31] : Outport  Port=4
  wires:
  C[t-1]/1 -> LSTM Cell[t=1]/1(C[t-1])
  h[t-1]/1 -> LSTM Cell[t=1]/2(h[t-1])
  LSTM Cell[t=1]/1(C[t]) -> LSTM Cell[t=2]/1(C[t-1])
  LSTM Cell[t=1]/2(h[t]) -> Y[t=0]/1, LSTM Cell[t=2]/2(h[t-1])
  X1[t=0]/1 -> LSTM Cell[t=1]/3(X1)
  X2[t=0]/1 -> LSTM Cell[t=1]/4(X2)
  X1[t=1]/1 -> LSTM Cell[t=2]/3(X1)
  X2[t=1]/1 -> LSTM Cell[t=2]/4(X2)
  LSTM Cell[t=2]/1(C[t]) -> LSTM Cell [t]/1(C[t-1])
  LSTM Cell[t=2]/2(h[t]) -> Y[t=1]/1, LSTM Cell [t]/2(h[t-1])
  LSTM Cell [t]/1(C[t]) -> LSTM Cell [t=31]/1(C[t-1])
  X2[t]/1 -> LSTM Cell [t]/4(X2)
  X1[t]/1 -> LSTM Cell [t]/3(X1)
  X1[t=31]/1 -> LSTM Cell [t=31]/3(X1)
  X2[t=31]/1 -> LSTM Cell [t=31]/4(X2)
  LSTM Cell [t=31]/2(h[t]) -> Y[t=31]/1
  LSTM Cell [t]/2(h[t]) -> Y[t]/1, LSTM Cell [t=31]/2(h[t-1])

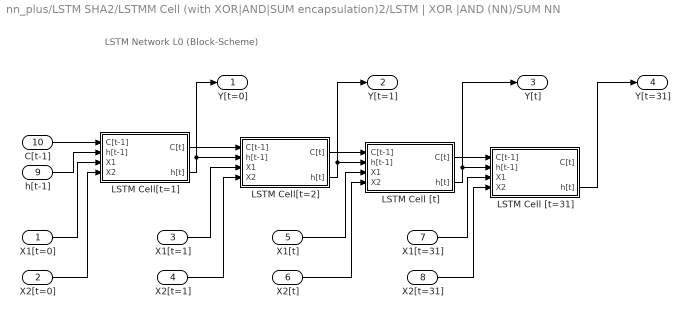
== system nn_plus/LSTM SHA2/LSTMM Cell (with XOR|AND|SUM encapsulation)2/LSTM | XOR |AND (NN)/SUM NN ==
  note: LSTM Network L0 (Block-Scheme)
  X1[t=0] : Inport
  X2[t=0] : Inport  Port=2
  X1[t=1] : Inport  Port=3
  X2[t=1] : Inport  Port=4
  X1[t] : Inport  Port=5
  X2[t] : Inport  Port=6
  X1[t=31] : Inport  Port=7
  X2[t=31] : Inport  Port=8
  h[t-1] : Inport  Port=9
  C[t-1] : Inport  Port=10
  LSTM Cell [t=31] : Subsystem
  LSTM Cell [t] : Subsystem
  LSTM Cell[t=1] : Subsystem
  LSTM Cell[t=2] : Subsystem
  Y[t=0] : Outport
  Y[t=1] : Outport  Port=2
  Y[t] : Outport  Port=3
  Y[t=31] : Outport  Port=4
  wires:
  C[t-1]/1 -> LSTM Cell[t=1]/1(C[t-1])
  h[t-1]/1 -> LSTM Cell[t=1]/2(h[t-1])
  LSTM Cell[t=1]/1(C[t]) -> LSTM Cell[t=2]/1(C[t-1])
  LSTM Cell[t=1]/2(h[t]) -> Y[t=0]/1, LSTM Cell[t=2]/2(h[t-1])
  X1[t=0]/1 -> LSTM Cell[t=1]/3(X1)
  X2[t=0]/1 -> LSTM Cell[t=1]/4(X2)
  X1[t=1]/1 -> LSTM Cell[t=2]/3(X1)
  X2[t=1]/1 -> LSTM Cell[t=2]/4(X2)
  LSTM Cell[t=2]/1(C[t]) -> LSTM Cell [t]/1(C[t-1])
  LSTM Cell[t=2]/2(h[t]) -> Y[t=1]/1, LSTM Cell [t]/2(h[t-1])
  LSTM Cell [t]/1(C[t]) -> LSTM Cell [t=31]/1(C[t-1])
  X2[t]/1 -> LSTM Cell [t]/4(X2)
  X1[t]/1 -> LSTM Cell [t]/3(X1)
  X1[t=31]/1 -> LSTM Cell [t=31]/3(X1)
  X2[t=31]/1 -> LSTM Cell [t=31]/4(X2)
  LSTM Cell [t=31]/2(h[t]) -> Y[t=31]/1
  LSTM Cell [t]/2(h[t]) -> Y[t]/1, LSTM Cell [t=31]/2(h[t-1])

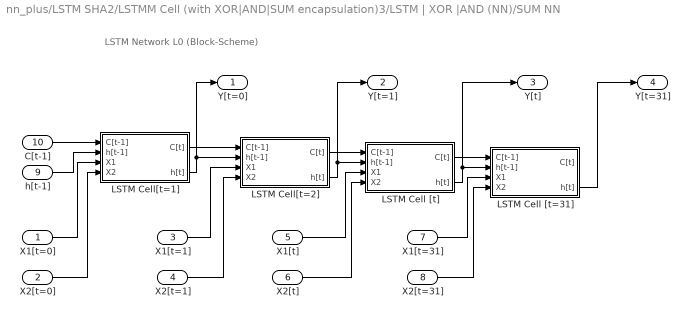
== system nn_plus/LSTM SHA2/LSTMM Cell (with XOR|AND|SUM encapsulation)3/LSTM | XOR |AND (NN)/SUM NN ==
  note: LSTM Network L0 (Block-Scheme)
  X1[t=0] : Inport
  X2[t=0] : Inport  Port=2
  X1[t=1] : Inport  Port=3
  X2[t=1] : Inport  Port=4
  X1[t] : Inport  Port=5
  X2[t] : Inport  Port=6
  X1[t=31] : Inport  Port=7
  X2[t=31] : Inport  Port=8
  h[t-1] : Inport  Port=9
  C[t-1] : Inport  Port=10
  LSTM Cell [t=31] : Subsystem
  LSTM Cell [t] : Subsystem
  LSTM Cell[t=1] : Subsystem
  LSTM Cell[t=2] : Subsystem
  Y[t=0] : Outport
  Y[t=1] : Outport  Port=2
  Y[t] : Outport  Port=3
  Y[t=31] : Outport  Port=4
  wires:
  C[t-1]/1 -> LSTM Cell[t=1]/1(C[t-1])
  h[t-1]/1 -> LSTM Cell[t=1]/2(h[t-1])
  LSTM Cell[t=1]/1(C[t]) -> LSTM Cell[t=2]/1(C[t-1])
  LSTM Cell[t=1]/2(h[t]) -> Y[t=0]/1, LSTM Cell[t=2]/2(h[t-1])
  X1[t=0]/1 -> LSTM Cell[t=1]/3(X1)
  X2[t=0]/1 -> LSTM Cell[t=1]/4(X2)
  X1[t=1]/1 -> LSTM Cell[t=2]/3(X1)
  X2[t=1]/1 -> LSTM Cell[t=2]/4(X2)
  LSTM Cell[t=2]/1(C[t]) -> LSTM Cell [t]/1(C[t-1])
  LSTM Cell[t=2]/2(h[t]) -> Y[t=1]/1, LSTM Cell [t]/2(h[t-1])
  LSTM Cell [t]/1(C[t]) -> LSTM Cell [t=31]/1(C[t-1])
  X2[t]/1 -> LSTM Cell [t]/4(X2)
  X1[t]/1 -> LSTM Cell [t]/3(X1)
  X1[t=31]/1 -> LSTM Cell [t=31]/3(X1)
  X2[t=31]/1 -> LSTM Cell [t=31]/4(X2)
  LSTM Cell [t=31]/2(h[t]) -> Y[t=31]/1
  LSTM Cell [t]/2(h[t]) -> Y[t]/1, LSTM Cell [t=31]/2(h[t-1])

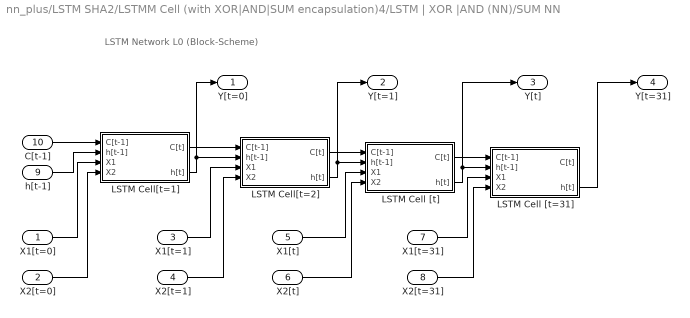
== system nn_plus/LSTM SHA2/LSTMM Cell (with XOR|AND|SUM encapsulation)4/LSTM | XOR |AND (NN)/SUM NN ==
  note: LSTM Network L0 (Block-Scheme)
  X1[t=0] : Inport
  X2[t=0] : Inport  Port=2
  X1[t=1] : Inport  Port=3
  X2[t=1] : Inport  Port=4
  X1[t] : Inport  Port=5
  X2[t] : Inport  Port=6
  X1[t=31] : Inport  Port=7
  X2[t=31] : Inport  Port=8
  h[t-1] : Inport  Port=9
  C[t-1] : Inport  Port=10
  LSTM Cell [t=31] : Subsystem
  LSTM Cell [t] : Subsystem
  LSTM Cell[t=1] : Subsystem
  LSTM Cell[t=2] : Subsystem
  Y[t=0] : Outport
  Y[t=1] : Outport  Port=2
  Y[t] : Outport  Port=3
  Y[t=31] : Outport  Port=4
  wires:
  C[t-1]/1 -> LSTM Cell[t=1]/1(C[t-1])
  h[t-1]/1 -> LSTM Cell[t=1]/2(h[t-1])
  LSTM Cell[t=1]/1(C[t]) -> LSTM Cell[t=2]/1(C[t-1])
  LSTM Cell[t=1]/2(h[t]) -> Y[t=0]/1, LSTM Cell[t=2]/2(h[t-1])
  X1[t=0]/1 -> LSTM Cell[t=1]/3(X1)
  X2[t=0]/1 -> LSTM Cell[t=1]/4(X2)
  X1[t=1]/1 -> LSTM Cell[t=2]/3(X1)
  X2[t=1]/1 -> LSTM Cell[t=2]/4(X2)
  LSTM Cell[t=2]/1(C[t]) -> LSTM Cell [t]/1(C[t-1])
  LSTM Cell[t=2]/2(h[t]) -> Y[t=1]/1, LSTM Cell [t]/2(h[t-1])
  LSTM Cell [t]/1(C[t]) -> LSTM Cell [t=31]/1(C[t-1])
  X2[t]/1 -> LSTM Cell [t]/4(X2)
  X1[t]/1 -> LSTM Cell [t]/3(X1)
  X1[t=31]/1 -> LSTM Cell [t=31]/3(X1)
  X2[t=31]/1 -> LSTM Cell [t=31]/4(X2)
  LSTM Cell [t=31]/2(h[t]) -> Y[t=31]/1
  LSTM Cell [t]/2(h[t]) -> Y[t]/1, LSTM Cell [t=31]/2(h[t-1])

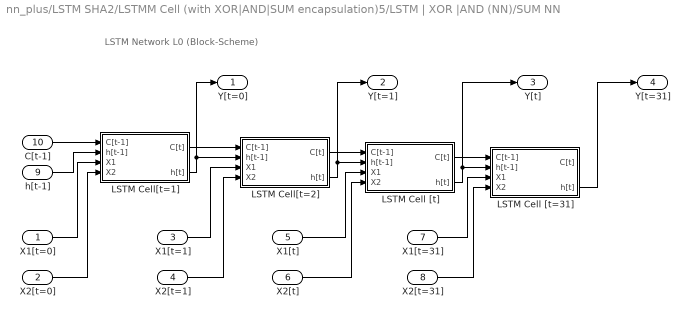
== system nn_plus/LSTM SHA2/LSTMM Cell (with XOR|AND|SUM encapsulation)5/LSTM | XOR |AND (NN)/SUM NN ==
  note: LSTM Network L0 (Block-Scheme)
  X1[t=0] : Inport
  X2[t=0] : Inport  Port=2
  X1[t=1] : Inport  Port=3
  X2[t=1] : Inport  Port=4
  X1[t] : Inport  Port=5
  X2[t] : Inport  Port=6
  X1[t=31] : Inport  Port=7
  X2[t=31] : Inport  Port=8
  h[t-1] : Inport  Port=9
  C[t-1] : Inport  Port=10
  LSTM Cell [t=31] : Subsystem
  LSTM Cell [t] : Subsystem
  LSTM Cell[t=1] : Subsystem
  LSTM Cell[t=2] : Subsystem
  Y[t=0] : Outport
  Y[t=1] : Outport  Port=2
  Y[t] : Outport  Port=3
  Y[t=31] : Outport  Port=4
  wires:
  C[t-1]/1 -> LSTM Cell[t=1]/1(C[t-1])
  h[t-1]/1 -> LSTM Cell[t=1]/2(h[t-1])
  LSTM Cell[t=1]/1(C[t]) -> LSTM Cell[t=2]/1(C[t-1])
  LSTM Cell[t=1]/2(h[t]) -> Y[t=0]/1, LSTM Cell[t=2]/2(h[t-1])
  X1[t=0]/1 -> LSTM Cell[t=1]/3(X1)
  X2[t=0]/1 -> LSTM Cell[t=1]/4(X2)
  X1[t=1]/1 -> LSTM Cell[t=2]/3(X1)
  X2[t=1]/1 -> LSTM Cell[t=2]/4(X2)
  LSTM Cell[t=2]/1(C[t]) -> LSTM Cell [t]/1(C[t-1])
  LSTM Cell[t=2]/2(h[t]) -> Y[t=1]/1, LSTM Cell [t]/2(h[t-1])
  LSTM Cell [t]/1(C[t]) -> LSTM Cell [t=31]/1(C[t-1])
  X2[t]/1 -> LSTM Cell [t]/4(X2)
  X1[t]/1 -> LSTM Cell [t]/3(X1)
  X1[t=31]/1 -> LSTM Cell [t=31]/3(X1)
  X2[t=31]/1 -> LSTM Cell [t=31]/4(X2)
  LSTM Cell [t=31]/2(h[t]) -> Y[t=31]/1
  LSTM Cell [t]/2(h[t]) -> Y[t]/1, LSTM Cell [t=31]/2(h[t-1])

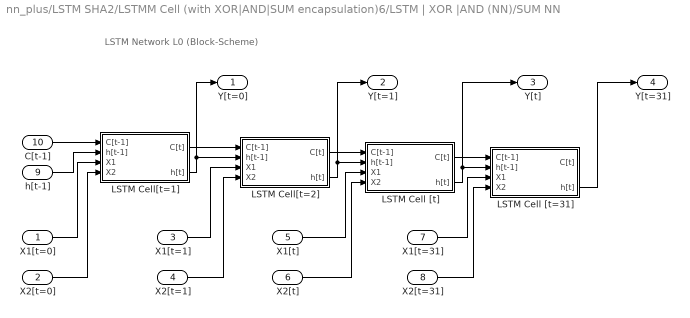
== system nn_plus/LSTM SHA2/LSTMM Cell (with XOR|AND|SUM encapsulation)6/LSTM | XOR |AND (NN)/SUM NN ==
  note: LSTM Network L0 (Block-Scheme)
  X1[t=0] : Inport
  X2[t=0] : Inport  Port=2
  X1[t=1] : Inport  Port=3
  X2[t=1] : Inport  Port=4
  X1[t] : Inport  Port=5
  X2[t] : Inport  Port=6
  X1[t=31] : Inport  Port=7
  X2[t=31] : Inport  Port=8
  h[t-1] : Inport  Port=9
  C[t-1] : Inport  Port=10
  LSTM Cell [t=31] : Subsystem
  LSTM Cell [t] : Subsystem
  LSTM Cell[t=1] : Subsystem
  LSTM Cell[t=2] : Subsystem
  Y[t=0] : Outport
  Y[t=1] : Outport  Port=2
  Y[t] : Outport  Port=3
  Y[t=31] : Outport  Port=4
  wires:
  C[t-1]/1 -> LSTM Cell[t=1]/1(C[t-1])
  h[t-1]/1 -> LSTM Cell[t=1]/2(h[t-1])
  LSTM Cell[t=1]/1(C[t]) -> LSTM Cell[t=2]/1(C[t-1])
  LSTM Cell[t=1]/2(h[t]) -> Y[t=0]/1, LSTM Cell[t=2]/2(h[t-1])
  X1[t=0]/1 -> LSTM Cell[t=1]/3(X1)
  X2[t=0]/1 -> LSTM Cell[t=1]/4(X2)
  X1[t=1]/1 -> LSTM Cell[t=2]/3(X1)
  X2[t=1]/1 -> LSTM Cell[t=2]/4(X2)
  LSTM Cell[t=2]/1(C[t]) -> LSTM Cell [t]/1(C[t-1])
  LSTM Cell[t=2]/2(h[t]) -> Y[t=1]/1, LSTM Cell [t]/2(h[t-1])
  LSTM Cell [t]/1(C[t]) -> LSTM Cell [t=31]/1(C[t-1])
  X2[t]/1 -> LSTM Cell [t]/4(X2)
  X1[t]/1 -> LSTM Cell [t]/3(X1)
  X1[t=31]/1 -> LSTM Cell [t=31]/3(X1)
  X2[t=31]/1 -> LSTM Cell [t=31]/4(X2)
  LSTM Cell [t=31]/2(h[t]) -> Y[t=31]/1
  LSTM Cell [t]/2(h[t]) -> Y[t]/1, LSTM Cell [t=31]/2(h[t-1])

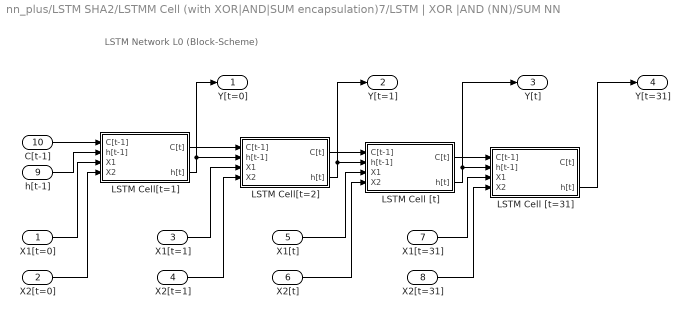
== system nn_plus/LSTM SHA2/LSTMM Cell (with XOR|AND|SUM encapsulation)7/LSTM | XOR |AND (NN)/SUM NN ==
  note: LSTM Network L0 (Block-Scheme)
  X1[t=0] : Inport
  X2[t=0] : Inport  Port=2
  X1[t=1] : Inport  Port=3
  X2[t=1] : Inport  Port=4
  X1[t] : Inport  Port=5
  X2[t] : Inport  Port=6
  X1[t=31] : Inport  Port=7
  X2[t=31] : Inport  Port=8
  h[t-1] : Inport  Port=9
  C[t-1] : Inport  Port=10
  LSTM Cell [t=31] : Subsystem
  LSTM Cell [t] : Subsystem
  LSTM Cell[t=1] : Subsystem
  LSTM Cell[t=2] : Subsystem
  Y[t=0] : Outport
  Y[t=1] : Outport  Port=2
  Y[t] : Outport  Port=3
  Y[t=31] : Outport  Port=4
  wires:
  C[t-1]/1 -> LSTM Cell[t=1]/1(C[t-1])
  h[t-1]/1 -> LSTM Cell[t=1]/2(h[t-1])
  LSTM Cell[t=1]/1(C[t]) -> LSTM Cell[t=2]/1(C[t-1])
  LSTM Cell[t=1]/2(h[t]) -> Y[t=0]/1, LSTM Cell[t=2]/2(h[t-1])
  X1[t=0]/1 -> LSTM Cell[t=1]/3(X1)
  X2[t=0]/1 -> LSTM Cell[t=1]/4(X2)
  X1[t=1]/1 -> LSTM Cell[t=2]/3(X1)
  X2[t=1]/1 -> LSTM Cell[t=2]/4(X2)
  LSTM Cell[t=2]/1(C[t]) -> LSTM Cell [t]/1(C[t-1])
  LSTM Cell[t=2]/2(h[t]) -> Y[t=1]/1, LSTM Cell [t]/2(h[t-1])
  LSTM Cell [t]/1(C[t]) -> LSTM Cell [t=31]/1(C[t-1])
  X2[t]/1 -> LSTM Cell [t]/4(X2)
  X1[t]/1 -> LSTM Cell [t]/3(X1)
  X1[t=31]/1 -> LSTM Cell [t=31]/3(X1)
  X2[t=31]/1 -> LSTM Cell [t=31]/4(X2)
  LSTM Cell [t=31]/2(h[t]) -> Y[t=31]/1
  LSTM Cell [t]/2(h[t]) -> Y[t]/1, LSTM Cell [t=31]/2(h[t-1])

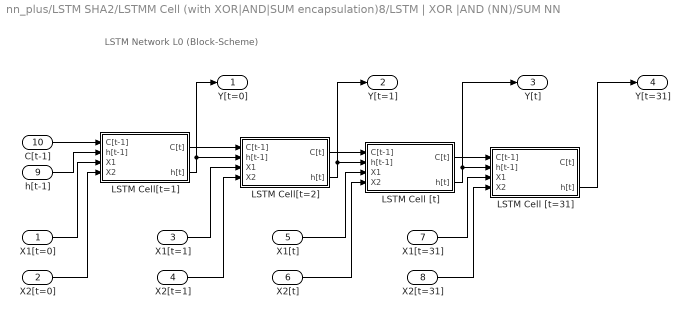
== system nn_plus/LSTM SHA2/LSTMM Cell (with XOR|AND|SUM encapsulation)8/LSTM | XOR |AND (NN)/SUM NN ==
  note: LSTM Network L0 (Block-Scheme)
  X1[t=0] : Inport
  X2[t=0] : Inport  Port=2
  X1[t=1] : Inport  Port=3
  X2[t=1] : Inport  Port=4
  X1[t] : Inport  Port=5
  X2[t] : Inport  Port=6
  X1[t=31] : Inport  Port=7
  X2[t=31] : Inport  Port=8
  h[t-1] : Inport  Port=9
  C[t-1] : Inport  Port=10
  LSTM Cell [t=31] : Subsystem
  LSTM Cell [t] : Subsystem
  LSTM Cell[t=1] : Subsystem
  LSTM Cell[t=2] : Subsystem
  Y[t=0] : Outport
  Y[t=1] : Outport  Port=2
  Y[t] : Outport  Port=3
  Y[t=31] : Outport  Port=4
  wires:
  C[t-1]/1 -> LSTM Cell[t=1]/1(C[t-1])
  h[t-1]/1 -> LSTM Cell[t=1]/2(h[t-1])
  LSTM Cell[t=1]/1(C[t]) -> LSTM Cell[t=2]/1(C[t-1])
  LSTM Cell[t=1]/2(h[t]) -> Y[t=0]/1, LSTM Cell[t=2]/2(h[t-1])
  X1[t=0]/1 -> LSTM Cell[t=1]/3(X1)
  X2[t=0]/1 -> LSTM Cell[t=1]/4(X2)
  X1[t=1]/1 -> LSTM Cell[t=2]/3(X1)
  X2[t=1]/1 -> LSTM Cell[t=2]/4(X2)
  LSTM Cell[t=2]/1(C[t]) -> LSTM Cell [t]/1(C[t-1])
  LSTM Cell[t=2]/2(h[t]) -> Y[t=1]/1, LSTM Cell [t]/2(h[t-1])
  LSTM Cell [t]/1(C[t]) -> LSTM Cell [t=31]/1(C[t-1])
  X2[t]/1 -> LSTM Cell [t]/4(X2)
  X1[t]/1 -> LSTM Cell [t]/3(X1)
  X1[t=31]/1 -> LSTM Cell [t=31]/3(X1)
  X2[t=31]/1 -> LSTM Cell [t=31]/4(X2)
  LSTM Cell [t=31]/2(h[t]) -> Y[t=31]/1
  LSTM Cell [t]/2(h[t]) -> Y[t]/1, LSTM Cell [t=31]/2(h[t-1])

== system nn_plus/LSTM SHA2/LSTMM Cell (with XOR|AND|SUM encapsulation)9/LSTM | XOR |AND (NN)/SUM NN ==
  note: LSTM Network L0 (Block-Scheme)
  X1[t=0] : Inport
  X2[t=0] : Inport  Port=2
  X1[t=1] : Inport  Port=3
  X2[t=1] : Inport  Port=4
  X1[t] : Inport  Port=5
  X2[t] : Inport  Port=6
  X1[t=31] : Inport  Port=7
  X2[t=31] : Inport  Port=8
  h[t-1] : Inport  Port=9
  C[t-1] : Inport  Port=10
  LSTM Cell [t=31] : Subsystem
  LSTM Cell [t] : Subsystem
  LSTM Cell[t=1] : Subsystem
  LSTM Cell[t=2] : Subsystem
  Y[t=0] : Outport
  Y[t=1] : Outport  Port=2
  Y[t] : Outport  Port=3
  Y[t=31] : Outport  Port=4
  wires:
  C[t-1]/1 -> LSTM Cell[t=1]/1(C[t-1])
  h[t-1]/1 -> LSTM Cell[t=1]/2(h[t-1])
  LSTM Cell[t=1]/1(C[t]) -> LSTM Cell[t=2]/1(C[t-1])
  LSTM Cell[t=1]/2(h[t]) -> Y[t=0]/1, LSTM Cell[t=2]/2(h[t-1])
  X1[t=0]/1 -> LSTM Cell[t=1]/3(X1)
  X2[t=0]/1 -> LSTM Cell[t=1]/4(X2)
  X1[t=1]/1 -> LSTM Cell[t=2]/3(X1)
  X2[t=1]/1 -> LSTM Cell[t=2]/4(X2)
  LSTM Cell[t=2]/1(C[t]) -> LSTM Cell [t]/1(C[t-1])
  LSTM Cell[t=2]/2(h[t]) -> Y[t=1]/1, LSTM Cell [t]/2(h[t-1])
  LSTM Cell [t]/1(C[t]) -> LSTM Cell [t=31]/1(C[t-1])
  X2[t]/1 -> LSTM Cell [t]/4(X2)
  X1[t]/1 -> LSTM Cell [t]/3(X1)
  X1[t=31]/1 -> LSTM Cell [t=31]/3(X1)
  X2[t=31]/1 -> LSTM Cell [t=31]/4(X2)
  LSTM Cell [t=31]/2(h[t]) -> Y[t=31]/1
  LSTM Cell [t]/2(h[t]) -> Y[t]/1, LSTM Cell [t=31]/2(h[t-1])

== system nn_plus/LSTM SHA2/LSTMM Cell (with XOR|AND|SUM encapsulation)/LSTM | XOR |AND (NN)/SUM NN/LSTM Cell [t=31] ==
  C[t-1] : Inport
  h[t-1] : Inport  Port=2
  X1 : Inport  Port=3
  X2 : Inport  Port=4
  Product : Product
  Product1 : Product
  Sum : Sum  Inputs=|++
  Sum1 : Sum  Inputs=|++
  Vector Concatenate : Concatenate  NumInputs=3
  logsig : neural/Transfer Functions/logsig
  logsig1 : neural/Transfer Functions/logsig
  logsig2 : neural/Transfer Functions/logsig
  tansig3 : neural/Transfer Functions/tansig
  tansig4 : neural/Transfer Functions/tansig
  C[t] : Outport
  h[t] : Outport  Port=2
  wires:
  h[t-1]/1 -> Vector Concatenate/1
  X1/1 -> Vector Concatenate/2
  X2/1 -> Vector Concatenate/3
  Vector Concatenate/1 -> tansig3/1, logsig2/1, logsig1/1, logsig/1
  C[t-1]/1 -> Sum/1
  logsig/1 -> Sum/2
  Sum/1 -> Sum1/1
  tansig3/1 -> Product/2
  logsig1/1 -> Product/1
  Product/1 -> Sum1/2
  logsig2/1 -> Product1/2
  Sum1/1 -> C[t]/1, tansig4/1
  tansig4/1 -> Product1/1
  Product1/1 -> h[t]/1

== system nn_plus/LSTM SHA2/LSTMM Cell (with XOR|AND|SUM encapsulation)/LSTM | XOR |AND (NN)/SUM NN/LSTM Cell [t] ==
  C[t-1] : Inport
  h[t-1] : Inport  Port=2
  X1 : Inport  Port=3
  X2 : Inport  Port=4
  Product : Product
  Product1 : Product
  Sum : Sum  Inputs=|++
  Sum1 : Sum  Inputs=|++
  Vector Concatenate : Concatenate  NumInputs=3
  logsig : neural/Transfer Functions/logsig
  logsig1 : neural/Transfer Functions/logsig
  logsig2 : neural/Transfer Functions/logsig
  tansig3 : neural/Transfer Functions/tansig
  tansig4 : neural/Transfer Functions/tansig
  C[t] : Outport
  h[t] : Outport  Port=2
  wires:
  h[t-1]/1 -> Vector Concatenate/1
  X1/1 -> Vector Concatenate/2
  X2/1 -> Vector Concatenate/3
  Vector Concatenate/1 -> tansig3/1, logsig2/1, logsig1/1, logsig/1
  C[t-1]/1 -> Sum/1
  logsig/1 -> Sum/2
  Sum/1 -> Sum1/1
  tansig3/1 -> Product/2
  logsig1/1 -> Product/1
  Product/1 -> Sum1/2
  logsig2/1 -> Product1/2
  Sum1/1 -> C[t]/1, tansig4/1
  tansig4/1 -> Product1/1
  Product1/1 -> h[t]/1

== system nn_plus/LSTM SHA2/LSTMM Cell (with XOR|AND|SUM encapsulation)/LSTM | XOR |AND (NN)/SUM NN/LSTM Cell[t=1] ==
  note: LSTM Cell L1 (Block-Scheme)
  C[t-1] : Inport
  h[t-1] : Inport  Port=2
  X1 : Inport  Port=3
  X2 : Inport  Port=4
  Product : Product
  Product1 : Product
  Sum : Sum  Inputs=|++
  Sum1 : Sum  Inputs=|++
  Vector Concatenate : Concatenate  NumInputs=3
  logsig : neural/Transfer Functions/logsig
  logsig1 : neural/Transfer Functions/logsig
  logsig2 : neural/Transfer Functions/logsig
  tansig3 : neural/Transfer Functions/tansig
  tansig4 : neural/Transfer Functions/tansig
  C[t] : Outport
  h[t] : Outport  Port=2
  wires:
  h[t-1]/1 -> Vector Concatenate/1
  X1/1 -> Vector Concatenate/2
  X2/1 -> Vector Concatenate/3
  Vector Concatenate/1 -> logsig/1, logsig2/1, tansig3/1, logsig1/1
  C[t-1]/1 -> Sum/1
  logsig/1 -> Sum/2
  Sum/1 -> Sum1/1
  tansig3/1 -> Product/2
  logsig1/1 -> Product/1
  Product/1 -> Sum1/2
  logsig2/1 -> Product1/2
  Sum1/1 -> C[t]/1, tansig4/1
  tansig4/1 -> Product1/1
  Product1/1 -> h[t]/1

== system nn_plus/LSTM SHA2/LSTMM Cell (with XOR|AND|SUM encapsulation)/LSTM | XOR |AND (NN)/SUM NN/LSTM Cell[t=2] ==
  C[t-1] : Inport
  h[t-1] : Inport  Port=2
  X1 : Inport  Port=3
  X2 : Inport  Port=4
  Product : Product
  Product1 : Product
  Sum : Sum  Inputs=|++
  Sum1 : Sum  Inputs=|++
  Vector Concatenate : Concatenate  NumInputs=3
  logsig : neural/Transfer Functions/logsig
  logsig1 : neural/Transfer Functions/logsig
  logsig2 : neural/Transfer Functions/logsig
  tansig3 : neural/Transfer Functions/tansig
  tansig4 : neural/Transfer Functions/tansig
  C[t] : Outport
  h[t] : Outport  Port=2
  wires:
  h[t-1]/1 -> Vector Concatenate/1
  X1/1 -> Vector Concatenate/2
  X2/1 -> Vector Concatenate/3
  Vector Concatenate/1 -> tansig3/1, logsig2/1, logsig1/1, logsig/1
  C[t-1]/1 -> Sum/1
  logsig/1 -> Sum/2
  Sum/1 -> Sum1/1
  tansig3/1 -> Product/2
  logsig1/1 -> Product/1
  Product/1 -> Sum1/2
  logsig2/1 -> Product1/2
  Sum1/1 -> C[t]/1, tansig4/1
  tansig4/1 -> Product1/1
  Product1/1 -> h[t]/1

== system nn_plus/LSTM SHA2/LSTMM Cell (with XOR|AND|SUM encapsulation)1/LSTM | XOR |AND (NN)/SUM NN/LSTM Cell [t=31] ==
  C[t-1] : Inport
  h[t-1] : Inport  Port=2
  X1 : Inport  Port=3
  X2 : Inport  Port=4
  Product : Product
  Product1 : Product
  Sum : Sum  Inputs=|++
  Sum1 : Sum  Inputs=|++
  Vector Concatenate : Concatenate  NumInputs=3
  logsig : neural/Transfer Functions/logsig
  logsig1 : neural/Transfer Functions/logsig
  logsig2 : neural/Transfer Functions/logsig
  tansig3 : neural/Transfer Functions/tansig
  tansig4 : neural/Transfer Functions/tansig
  C[t] : Outport
  h[t] : Outport  Port=2
  wires:
  h[t-1]/1 -> Vector Concatenate/1
  X1/1 -> Vector Concatenate/2
  X2/1 -> Vector Concatenate/3
  Vector Concatenate/1 -> tansig3/1, logsig2/1, logsig1/1, logsig/1
  C[t-1]/1 -> Sum/1
  logsig/1 -> Sum/2
  Sum/1 -> Sum1/1
  tansig3/1 -> Product/2
  logsig1/1 -> Product/1
  Product/1 -> Sum1/2
  logsig2/1 -> Product1/2
  Sum1/1 -> C[t]/1, tansig4/1
  tansig4/1 -> Product1/1
  Product1/1 -> h[t]/1
